simulink model "omni_server_2"  (Simulink 7.0)
settings: Solver=ode1  StartTime=0.0  StopTime=inf  FixedStep=0.001  RelTol=1e-3
libraries: quarc_library x2, simulink x1
settings Model: Creator=colinlea  LastModifiedBy=colinlea  SimulationMode=external  ExtModeTrigDuration=10000
settings SolverCC: PositivePriorityOrder=on
settings RTWCC: SystemTargetFile=quarc_windows.tlc  TemplateMakefile=quarc_default_tmf  Description=QuaRC Win32 Target  ProcessScript=quarc_windows_make_rtw_hook
settings STFCustomTargetCC: TargetPreCompLibLocation=C:\DOCUME~1\ALLUSE~1\APPLIC~1\QuaRC\lib\2007b\windows\release  GenFloatMathFcnCalls=ANSI_C  SystemTargetFile=quarc_windows.tlc
settings GRTTargetCC: TargetPreCompLibLocation=C:\DOCUME~1\ALLUSE~1\APPLIC~1\QuaRC\lib\2007b\windows\release  CompOptLevelCompliant=off  MatFileLogging=off  ExtMode=on  ExtModeMexFile=quarc_comm

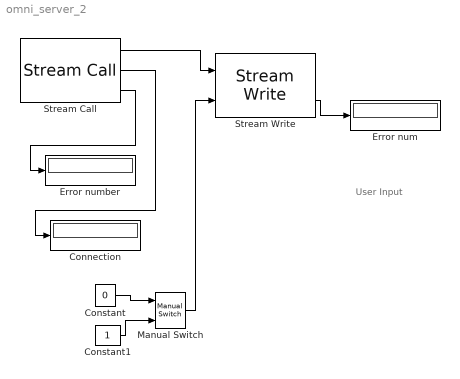
== system omni_server_2 ==
  note: User Input
  Connection : Display
  Constant : Constant  Value=0  OutDataType=sfix(16)  OutScaling=2^0
  Constant1 : Constant  OutDataType=sfix(16)  OutScaling=2^0
  Error num : Display
  Error number : Display
  Manual Switch : simulink/Signal Routing/Manual Switch  SystemSampleTime=-1  sw=0  action=0  varsize=off
  Stream Call : quarc_library/Communications/Intermediate/Stream Call  uri_source=Internal (dialog parameter)  uri=tcpip://localhost:18002  send_buffer_size=8000  receive_buffer_size=8000  byte_order=little endian (Intel - LSB first)  sample_time=qc_get_step_size  active=off
      settings: AttributesFormatString=(%<uri>)
  Stream Write : quarc_library/Communications/Intermediate/Stream Write  optimization=Minimizing latency
  wires:
  Stream Call/2 -> Connection/1
  Stream Call/3 -> Error number/1
  Stream Write/2 -> Error num/1
  Manual Switch/1 -> Stream Write/2
  Constant/1 -> Manual Switch/1
  Constant1/1 -> Manual Switch/2
  Stream Call/1 -> Stream Write/1
